simulink model "sampleModel1780"  (R2023a)
settings: Solver=VariableStepAuto  StartTime=0.0  StopTime=10.0  RelTol=1e-3
libraries: hdlsllib x5
settings Model: Creator=user1  LastModifiedBy=user1

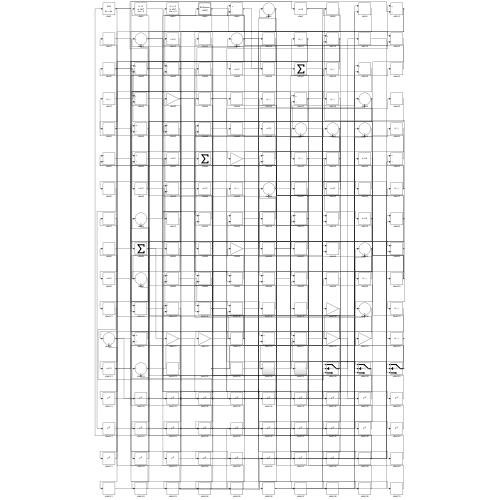
[thumbnail: Simulink's stored preview of the top-level diagram]
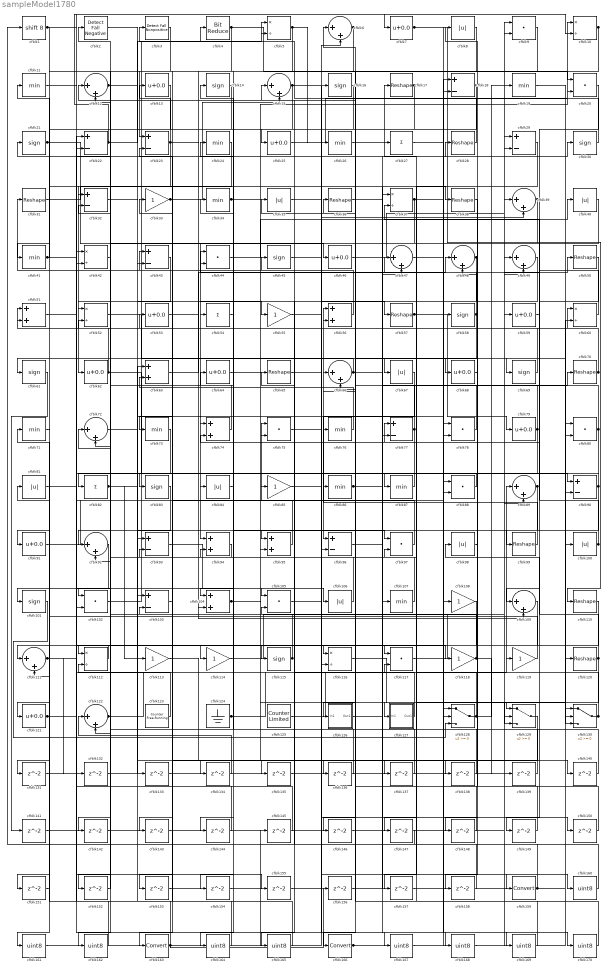
== system sampleModel1780 ==
  cfblk1 : ArithShift  BitShiftNumber=8
  cfblk{5,10,37,42,52,60,112,116} (8 alike) : Product  Inputs=*/  RndMeth=Zero  SaturateOnIntegerOverflow=on
  cfblk{8,35,40,67,81,84,98,100,106} (9 alike) : Abs  SaturateOnIntegerOverflow=off
  cfblk{14,16,21,30,45,58,61,69,83,101,115} (11 alike) : Signum
  cfblk{9,20,44,75,78,80,88,97,102,105,117} (11 alike) : DotProduct  OutDataTypeStr=Inherit: Inherit via internal rule
  cfblk{18,22..23,29,32,43,77,90,93,96,103} (11 alike) : Sum  Inputs=+-
  cfblk{51,56,63,74,94..95,104} (7 alike) : Sum
  cfblk{11,19,24,26,34,41,71,73,76,86..87,107} (12 alike) : MinMax
  cfblk{33,55,85,108,113..114,118..119} (8 alike) : Gain
  cfblk{6,12,15,39,47..49,66,72,89,92,109,111,122} (14 alike) : Sum  Inputs=|++
  cfblk{17,28,31,36,38,50,57,65,70,99,110,120} (12 alike) : Reshape
  cfblk{7,13,25,46,53,59,62,64,68,79,91,121} (12 alike) : Bias  Bias=0.0  SaturateOnIntegerOverflow=off
  cfblk123 : hdlsllib/Sources/Counter Free-Running  NumBits=16  tsamp=-1
  cfblk124 : Ground
  cfblk125 : hdlsllib/Sources/Counter Limited  uplimit=7  tsamp=-1
  cfblk126 : Subsystem
      settings: LibrarySourceBlock=|
      | hdlsllib/Ports &
      | Subsystems/Subsystem
  cfblk127 : Subsystem
      settings: LibrarySourceBlock=|
      | hdlsllib/Ports &
      | Subsystems/Subsystem
  cfblk128 : Switch  SaturateOnIntegerOverflow=off  InputSameDT=off
  cfblk129 : Switch  SaturateOnIntegerOverflow=off  InputSameDT=off
  cfblk130 : Switch  SaturateOnIntegerOverflow=off  InputSameDT=off
  cfblk{131..158} (28 alike) : Delay  SampleTime=1
  cfblk159 : DataTypeConversion  SaturateOnIntegerOverflow=off  RndMeth=Floor
  cfblk{160..162,164..165,167..170} (9 alike) : DataTypeConversion  OutDataTypeStr=uint8  SaturateOnIntegerOverflow=off  RndMeth=Floor
  cfblk163 : DataTypeConversion  SaturateOnIntegerOverflow=off  RndMeth=Floor
  cfblk166 : DataTypeConversion  SaturateOnIntegerOverflow=off  RndMeth=Floor
  cfblk2 : hdlsllib/Logic and Bit Operations/Detect Fall Negative  vinit=0  OutDataTypeStr=boolean
  cfblk27 : Sum  Inputs=+
  cfblk3 : hdlsllib/Logic and Bit Operations/Detect Fall Nonpositive  vinit=0  OutDataTypeStr=boolean
  cfblk4 : hdlsllib/Logic and Bit Operations/Bit Reduce  mode=AND
  cfblk54 : Sum  Inputs=+
  cfblk82 : Sum  Inputs=+
  wires:
  cfblk102/1 -> cfblk4/1
  cfblk112/1 -> cfblk111/1
  cfblk60/1 -> cfblk94/1
  cfblk21/1 -> cfblk46/1, cfblk107/1
  cfblk7/1 -> cfblk110/1, cfblk90/2
  cfblk56/1 -> cfblk31/1
  cfblk100/1 -> cfblk44/1, cfblk74/2, cfblk37/2
  cfblk80/1 -> cfblk96/1, cfblk51/1, cfblk52/2, cfblk130/3
  cfblk115/1 -> cfblk64/1, cfblk72/2
  cfblk79/1 -> cfblk12/1, cfblk164/1
  cfblk93/1 -> cfblk105/1
  cfblk22/1 -> cfblk7/1, cfblk95/1, cfblk5/2
  cfblk99/1 -> cfblk56/1
  cfblk130/1 -> cfblk89/1, cfblk77/1
  cfblk127/1(Out1) -> cfblk45/1
  cfblk70/1 -> cfblk60/1, cfblk56/2
  cfblk34/1 -> cfblk20/2, cfblk137/1
  cfblk67/1 -> cfblk86/1
  cfblk3/1 -> cfblk101/1
  cfblk111/1 -> cfblk132/1, cfblk170/1
  cfblk63/1 -> cfblk48/1
  cfblk58/1 -> cfblk15/1, cfblk116/1
  cfblk88/1 -> cfblk82/1
  cfblk8/1 -> cfblk23/1
  cfblk4/1 -> cfblk108/1, cfblk153/1
  cfblk82/1 -> cfblk113/1, cfblk135/1
  cfblk107/1 -> cfblk43/1
  cfblk90/1 -> cfblk84/1, cfblk117/1
  cfblk62/1 -> cfblk87/1, cfblk51/2
  cfblk124/1 -> cfblk88/1, cfblk18/2
  cfblk43/1 -> cfblk112/1
  cfblk52/1 -> cfblk120/1
  cfblk118/1 -> cfblk65/1, cfblk34/1, cfblk139/1
  cfblk39/1 -> cfblk104/1, cfblk68/1
  cfblk10/1 -> cfblk73/1, cfblk154/1
  cfblk119/1 -> cfblk81/1
  cfblk125/1 -> cfblk119/1
  cfblk65/1 -> cfblk88/2
  cfblk91/1 -> cfblk18/1
  cfblk26/1 -> cfblk17/1
  cfblk19/1 -> cfblk100/1
  cfblk23/1 -> cfblk62/1, cfblk13/1, cfblk109/2
  cfblk97/1 -> cfblk33/1
  cfblk57/1 -> cfblk79/1, cfblk157/1
  cfblk72/1 -> cfblk74/1
  cfblk103/1 -> cfblk163/1
  cfblk28/1 -> cfblk5/1
  cfblk66/1 -> cfblk61/1, cfblk130/2
  cfblk122/1 -> cfblk2/1, cfblk59/1
  cfblk55/1 -> cfblk39/2
  cfblk44/1 -> cfblk40/1
  cfblk35/1 -> cfblk57/1
  cfblk18/1 -> cfblk83/1, cfblk22/2
  cfblk114/1 -> cfblk29/2
  cfblk85/1 -> cfblk16/1
  cfblk20/1 -> cfblk109/1
  cfblk117/1 -> cfblk50/1
  cfblk29/1 -> cfblk67/1
  cfblk84/1 -> cfblk14/1
  cfblk12/1 -> cfblk55/1, cfblk134/1
  cfblk33/1 -> cfblk15/2, cfblk95/2
  cfblk16/1 -> cfblk43/2
  cfblk40/1 -> cfblk92/1
  cfblk104/1 -> cfblk118/1, cfblk140/1
  cfblk48/1 -> cfblk54/1, cfblk165/1
  cfblk73/1 -> cfblk102/1
  cfblk92/1 -> cfblk121/1
  cfblk37/1 -> cfblk129/3, cfblk142/1
  cfblk68/1 -> cfblk8/1
  cfblk126/1(Out1) -> cfblk37/1
  cfblk31/1 -> cfblk38/1
  cfblk14/1 -> cfblk52/1
  cfblk42/1 -> cfblk122/2
  cfblk77/1 -> cfblk53/1, cfblk75/2
  cfblk116/1 -> cfblk129/1
  cfblk120/1 -> cfblk98/1, cfblk147/1
  cfblk53/1 -> cfblk97/1
  cfblk64/1 -> cfblk127/1(In1)
  cfblk46/1 -> cfblk9/1
  cfblk25/1 -> cfblk10/1
  cfblk47/1 -> cfblk69/1
  cfblk1/1 -> cfblk106/1, cfblk10/2, cfblk41/1
  cfblk11/1 -> cfblk115/1
  cfblk36/1 -> cfblk159/1
  cfblk13/1 -> cfblk102/2
  cfblk9/1 -> cfblk76/1
  cfblk74/1 -> cfblk12/2
  cfblk41/1 -> cfblk11/1, cfblk90/1
  cfblk5/1 -> cfblk104/2, cfblk26/1
  cfblk76/1 -> cfblk63/2
  cfblk54/1 -> cfblk114/1
  cfblk69/1 -> cfblk24/1
  cfblk6/1 -> cfblk32/1, cfblk42/2
  cfblk95/1 -> cfblk75/1
  cfblk94/1 -> cfblk93/2
  cfblk123/1 -> cfblk32/2
  cfblk86/1 -> cfblk70/1, cfblk47/2
  cfblk81/1 -> cfblk28/1
  cfblk17/1 -> cfblk25/1, cfblk151/1
  cfblk30/1 -> cfblk3/1
  cfblk15/1 -> cfblk91/1, cfblk20/1, cfblk129/2
  cfblk2/1 -> cfblk78/2
  cfblk49/1 -> cfblk166/1
  cfblk121/1 -> cfblk85/1, cfblk117/2
  cfblk89/1 -> cfblk126/1(In1), cfblk144/1
  cfblk96/1 -> cfblk30/1
  cfblk101/1 -> cfblk128/3
  cfblk78/1 -> cfblk35/1
  cfblk128/1 -> cfblk47/1, cfblk19/1
  cfblk106/1 -> cfblk21/1
  cfblk59/1 -> cfblk99/1
  cfblk87/1 -> cfblk66/2
  cfblk24/1 -> cfblk131/1
  cfblk131/1 -> cfblk128/2
  cfblk132/1 -> cfblk29/1
  cfblk32/1 -> cfblk133/1
  cfblk133/1 -> cfblk6/2
  cfblk134/1 -> cfblk122/1
  cfblk135/1 -> cfblk128/1
  cfblk113/1 -> cfblk136/1
  cfblk136/1 -> cfblk93/1
  cfblk137/1 -> cfblk94/2
  cfblk109/1 -> cfblk138/1
  cfblk138/1 -> cfblk63/1
  cfblk139/1 -> cfblk44/2
  cfblk140/1 -> cfblk92/2
  cfblk61/1 -> cfblk141/1
  cfblk141/1 -> cfblk9/2
  cfblk142/1 -> cfblk89/2
  cfblk129/1 -> cfblk143/1
  cfblk143/1 -> cfblk96/2
  cfblk144/1 -> cfblk23/2
  cfblk145/1 -> cfblk42/1
  cfblk110/1 -> cfblk146/1
  cfblk147/1 -> cfblk1/1
  cfblk98/1 -> cfblk148/1
  cfblk148/1 -> cfblk97/2
  cfblk50/1 -> cfblk149/1
  cfblk149/1 -> cfblk66/1
  cfblk75/1 -> cfblk150/1
  cfblk150/1 -> cfblk48/2
  cfblk151/1 -> cfblk111/2
  cfblk108/1 -> cfblk152/1
  cfblk152/1 -> cfblk112/2
  cfblk153/1 -> cfblk130/1
  cfblk154/1 -> cfblk77/2
  cfblk51/1 -> cfblk155/1
  cfblk155/1 -> cfblk39/1
  cfblk156/1 -> cfblk60/2
  cfblk157/1 -> cfblk80/2
  cfblk38/1 -> cfblk158/1
  cfblk158/1 -> cfblk105/2
  cfblk159/1 -> cfblk72/1, cfblk78/1
  cfblk45/1 -> cfblk160/1
  cfblk160/1 -> cfblk36/1
  cfblk71/1 -> cfblk161/1
  cfblk161/1 -> cfblk145/1
  cfblk83/1 -> cfblk162/1
  cfblk162/1 -> cfblk71/1
  cfblk163/1 -> cfblk156/1, cfblk116/2, cfblk22/1
  cfblk164/1 -> cfblk103/1
  cfblk165/1 -> cfblk103/2
  cfblk166/1 -> cfblk58/1, cfblk80/1
  cfblk105/1 -> cfblk167/1
  cfblk167/1 -> cfblk49/1
  cfblk146/1 -> cfblk168/1
  cfblk168/1 -> cfblk49/2
  cfblk27/1 -> cfblk169/1
  cfblk169/1 -> cfblk6/1
  cfblk170/1 -> cfblk27/1

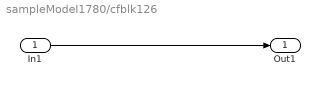
== system sampleModel1780/cfblk126 ==
  In1 : Inport
  Out1 : Outport
  wires:
  In1/1 -> Out1/1

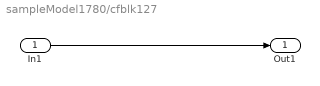
== system sampleModel1780/cfblk127 ==
  In1 : Inport
  Out1 : Outport
  wires:
  In1/1 -> Out1/1
